simulink model "VCMGCM1962020b_v2"  (R2020b)
settings: Solver=FixedStepDiscrete  StartTime=0.0  StopTime=10.0  FixedStep=0.005  RelTol=1e-3  EnableMultiTasking=on
PreLoadFcn:
  | try, model_open; catch, disp('Error occurred while executing model pre-load callback: model_open.m'); disp('Please assure that the MATLAB working directory is set to the model directory before opening.'); end
InitFcn:
  | try, model_open; catch, end
undefined symbols (not defined in the file): Bridge, GCM, H, raptor_get_param_eval, raptor_get_safe_string, raptor_xcp_function
libraries: Blocks_lib x1165, Raptor_lib x665, simulink x62, VCM_lib x5
(part 23 of 23)

== stateflow chart VCMGCM1962020b_v2/Fgnd/Actuators/CAN/Drive Inverter/NMT Sequence ==
  state Init
    en: NMTStep= 1
    en:tmr=0;
    tmr++;
  state NMTSequenceActive
    state NMTStep2
      en: NMTStep= 2
      en: tmr = 0;
      du: tmr++;
    state NMTStep3
      en: NMTStep= 3
      en: tmr = 0;
      du: tmr++;
    state NMTStep4
      en: NMTStep= 4
      en: tmr = 0;
      du: tmr++;
    state NMTStep8
      en: NMTStep= 8;en: tmr = 0;
      du: tmr++;
    state NMTStep5
      en: NMTStep= 5;en: tmr = 0;
      du: tmr++;
    state NMTStep6
      en: NMTStep= 6;en: tmr = 0;
      du: tmr++;
    state NMTStep7
      en: NMTStep= 7;en: tmr = 0;
      du: tmr++;
    NMTStep8 -> NMTStep2 : [RunMode]
    NMTStep2 -> NMTStep5 [order 1] : [AutoStrEnbl && HV_On&& RunMode]
    NMTStep2 -> NMTStep3 [order 2] : [HV_On && tmr>NMTStateDly ]
    NMTStep3 -> NMTStep4 : [tmr>  NMTStateDly]
    NMTStep4 -> NMTStep5 : [tmr>  NMTStateDly && RunMode]
    NMTStep7 -> NMTStep8 : [tmr>  NMTStateDly]
    NMTStep5 -> NMTStep6 : [tmr>  NMTStateDly && !RunMode]
    NMTStep6 -> NMTStep7 : [tmr > NoComTm]
  note: Step2:
      | Nothing sent Wait HV
      | Step3:
      | VCU1_StateCmd = 0x0 (Off)
      | VCU2_EmTorqDmd = 0 Nm
      | VCU2_EmVelDmd = 0 Nm
      | Step4(1Frame):
      | NMT_StateDms_0x01 (operational)
      | TargetNode = 0x01
      | Step5 :
      | Enable Run mode, and apply torque
      | VCU1_StateCmd = 0x1 (RUN)
      | Step6:
      | VCU1_StateCmd = 0x0 (OFF)
      | Step7:
      | NMT_StateDmd = 0x02 (STOP)
      | NMT_TargetNode = 0x01
      | 1 frame
      | Step8: Stop VCU1/2 transmit
      |
      | Step 10: Error Reset
  state ErrorState
    en: NMTStep= 10
    en: tmr = 0;
    du: tmr++;
  note: Error reset
  (default) -> Init
  Init -> NMTStep2 : [tmr>NMTStateDly && InvrtrEnble]
  NMTSequenceActive -> Init [order 2] : [!InvrtrEnble]
  ErrorState -> NMTStep3 : [tmr>  NMTStateDly]
  NMTSequenceActive -> ErrorState [order 1] : [EM1StateAct==2 || (!EMxRcved && tmr > NoComTm)]
  data: tmr local double; NMTStateDly input double; EMxRcved input boolean; NoComTm input; HV_On input uint8 size=1; RunMode input boolean; NMTStep output uint8; EM1StateAct input boolean; InvrtrEnble input boolean; AutoStrEnbl input boolean

== stateflow chart VCMGCM1962020b_v2/Fgnd/Control/Other/Heater/Heater Pump ==
  state PUMP_ON
    en: Pump = 1
    state HEATER_ON
    state HEATER_OFF
      en: Tmr = 1
      du: Tmr ++
      ex: Tmr = 1
    (default) -> HEATER_ON
    HEATER_ON -> HEATER_OFF : [ !Heater ]
    HEATER_OFF -> HEATER_ON : [ Heater ]
  state PUMP_OFF
    en: Pump = 0
  (default) -> PUMP_OFF
  PUMP_OFF -> PUMP_ON : [ Enbl && Heater ]
  PUMP_ON -> PUMP_OFF : [ !Enbl || ...
      |   Tmr >= HoldTime ]
  data: Enbl input; Pump output boolean size=1; Tmr local uint16 size=1; Heater input; HoldTime input

== stateflow chart VCMGCM1962020b_v2/Fgnd/Control/PDU/High-Voltage Discharge Contactor/HV Discharge ==
  state ENABLE
    state DISCHARGE
      en: Cntr = 1
      en: Tmr = 1
      du: Tmr ++
    state FAULT
      en: Cntr = 0
      en: EvalDiag(1)
      en: Tmr = 1
      du: Tmr ++
    (default) -> DISCHARGE
    DISCHARGE -> FAULT : [ Tmr >= MxTime ]
    FAULT -> DISCHARGE : [ Tmr >= RetryWaitTime ]
  state DISABLE
    en: Cntr = 0
  state EvalDiag(status) [function]
  (default) -> DISABLE
  DISABLE -> ENABLE : [ Enbl ]
  ENABLE -> DISABLE : [ !Enbl ]
      | { EvalDiag(0) }
  data: status function_input; Cntr output boolean size=1; Tmr local uint16 size=1; Enbl input; MxTime input; RetryWaitTime input

== stateflow chart VCMGCM1962020b_v2/Fgnd/Control/Other/Other/FMWS/Chart ==
  (junction 11) -> (junction 13) : {FMWS_State_gear = 194 }
  (junction 3) -> (junction 11) [order 1] : [Drv == 1]
  (junction 25) -> (junction 3)
  (junction 3) -> (junction 15) [order 2] : [Ntrl == 1]
  (junction 15) -> (junction 17) : {FMWS_State_gear = 192 }
  (junction 44) -> (junction 25) [order 1] : [PrkBrk == 0]
  (junction 3) -> (junction 21) [order 3] : [Rev ==1]
  (junction 21) -> (junction 19) : {FMWS_State_gear = 196}
  (junction 30) -> (junction 36) : {FMWS_State_gear = 146 }
  (default) -> (junction 44)
  (junction 32) -> (junction 30) [order 1] : [Drv == 1]
  (junction 44) -> (junction 29) [order 2] : [PrkBrk ==1]
  (junction 29) -> (junction 32)
  (junction 32) -> (junction 40) [order 2] : [Ntrl == 1]
  (junction 40) -> (junction 39) : {FMWS_State_gear = 144 }
  (junction 32) -> (junction 43) [order 3] : [Rev ==1]
  (junction 43) -> (junction 42) : {FMWS_State_gear = 148}
  data: Drv input; Ntrl input; Rev input; PrkBrk input; FMWS_State_gear output

== stateflow chart VCMGCM1962020b_v2/Fgnd/Actuators/CAN/Charger/Config Msgs/Config Sequence/Config Sequence ==
  state WAIT
  state CONFIG
    en: Tmr1 = 1
    du: Tmr1 ++
    state TX617_A5
      en: Tx617_A5
      en: Tmr2 = 1
      du: Tmr2 ++
    state TX617_00
      en: Tx617_00
    (default) -> TX617_A5
    (junction 80) -> TX617_A5
    (junction 71) -> (junction 80)
    TX617_A5 -> (junction 69) : [ Tmr2 >= TxRate ]
    (junction 69) -> (junction 71) [order 2]
    (junction 69) -> TX617_00 [order 1] : [ ConfigComplete ]
  (default) -> WAIT
  WAIT -> CONFIG : [ hasChangedTo(ConfigPrompt, 1) ]
  CONFIG -> WAIT : [ Tmr1 >= MxTime ]
  TX617_00 -> WAIT
  data: ConfigPrompt input; ConfigComplete input; Tmr1 local uint16 size=1; Tmr2 local uint16 size=1; MxTime input; TxRate input
  events: Tx617_A5 output FUNCTION_CALL_EVENT; Tx617_00 output FUNCTION_CALL_EVENT

== stateflow chart VCMGCM1962020b_v2/Fgnd/Control/Modes/PRND Mode/PRND_Act ==
  (junction 5) -> (junction 17) : {PRND_Act_Out = 25}
  (junction 3) -> (junction 5) [order 1] : [PRND_In == 0]
  (junction 6) -> (junction 13) : {PRND_Act_Out = -125}
  (junction 3) -> (junction 6) [order 2] : [PRND_In == 1]
  (default) -> (junction 3)
  (junction 3) -> (junction 7) [order 3] : [PRND_In == 3]
  (junction 3) -> (junction 8) [order 4] : [PRND_In == 2]
  (junction 7) -> (junction 15) : {PRND_Act_Out = 125}
  (junction 8) -> (junction 19) : {PRND_Act_Out = 125}
  data: PRND_In input; PRND_Act_Out output

== stateflow chart VCMGCM1962020b_v2/Fgnd/Actuators/CAN/CCS Interface/Commands/Commands ==
  state WAIT_FOR_CABLE
    en: Step = 0.00
    en: Command = 2 %Standby
    en: EVTargetVoltage = 0
    en: EVTargetCurrent = 0
    en: DCChgCntr = 0
    en: DC_ContactorsState = 0
    en: BattIsoTestDsbl = 0
    en: ChgPortDCVoltHiDiagEnbl = 1
  state ON_BOARD_AC_CHARGING
    state NO_FAULT
      state CHARGING
        state WAIT_FOR_READY_TO_CHARGE
          en: Step = 1.00
          en: Command = 3 %Start
        state CHARGING
          en: Step = 1.01
          en: Command = 5 %Charge
        (default) -> WAIT_FOR_READY_TO_CHARGE
        WAIT_FOR_READY_TO_CHARGE -> ON_BOARD_AC_CHARGING.NO_FAULT.CHARGING.CHARGING : [ CurrentState == 8 ]
            | %Active_Ready To Charge
      state END_CHARGE
        en: Step = 1.02
        en: Command = 6 %End Charge
      (default) -> ON_BOARD_AC_CHARGING.NO_FAULT.CHARGING
      ON_BOARD_AC_CHARGING.NO_FAULT.CHARGING -> ON_BOARD_AC_CHARGING.NO_FAULT.END_CHARGE : [ !ChgMode ]
    state FAULT
      en: Step = 1.03
      en: Command = 2 %Standby
    (default) -> ON_BOARD_AC_CHARGING.NO_FAULT
    ON_BOARD_AC_CHARGING.NO_FAULT -> ON_BOARD_AC_CHARGING.FAULT : [ CurrentState == 12 ]
        | %Fault
    ON_BOARD_AC_CHARGING.FAULT -> (junction 265) : [ CurrentState == 0 || ...
        |   CurrentState == 1 || ...
        |   CurrentState == 15 || ...
        |   CurrentState == 16 || ...
        |   CurrentState == 17 ]
        | %Standby_*
    ON_BOARD_AC_CHARGING.NO_FAULT.END_CHARGE -> (junction 264) : [ CurrentState == 0 || ...
        |   CurrentState == 1 || ...
        |   CurrentState == 15 || ...
        |   CurrentState == 16 || ...
        |   CurrentState == 17 ]
        | %Standby_*
    (junction 265) -> (junction 264)
  state OFF_BOARD_DC_CHARGING
    state NO_FAULT
      state EVSE_PRECHARGE_AND_CHARGING
        state WAIT_FOR_READY_TO_PRECHARGE
          en: Step = 2.00
          en: Command = 3 %Start
        state PRECHARGE
          en: Step = 2.01
          en: Command = 4 %PreCharge
          en, du: EVTargetVoltage = HVBusVolt
          en: EVTargetCurrent = EVTargetCurrentPreChg
          en: ChgPortDCVoltHiDiagEnbl = 0
        state EVSE_PRECHARGED
          en: Step = 2.02
          en: Command = 5 %Charge
          en, du: EVTargetVoltage = HVBusVolt
          en: BattIsoTestDsbl = 1
          en: Tmr = 1; du: Tmr ++
        state CLOSE_DC_CHARGE_CONTACTORS
          en: Step = 2.03
          en: DCChgCntr = 1
          en, du: EVTargetVoltage = HVBusVolt
        state WAIT_FOR_ACTIVE_CHARGING
          en: Step = 2.04
          en: DC_ContactorsState = 1
        state RAMP_IN_CURRENT
          en: Step = 2.05
          en: EVTargetVoltage = ChgrDCVoltSetpt
          du: EVTargetCurrent = ...
          EVTargetCurrent + EVTargetCurrentRampInRate
        state NORMAL_CHARGING
          en: Step = 2.06
          en, du: EVTargetCurrent = ChgrDCCurLim
        (default) -> WAIT_FOR_READY_TO_PRECHARGE
        WAIT_FOR_READY_TO_PRECHARGE -> PRECHARGE : [ CurrentState == 6 ]
            | %Active_Ready for PreCharge
        PRECHARGE -> EVSE_PRECHARGED : [ ChgPortDCVoltMatch ]
        EVSE_PRECHARGED -> CLOSE_DC_CHARGE_CONTACTORS : [ ChgPortDCVoltMatch && ...
            |   DC_CloseContactorsRequest && ...
            |   Tmr >= BattIsoTestDsblTime ]
        CLOSE_DC_CHARGE_CONTACTORS -> WAIT_FOR_ACTIVE_CHARGING : [ DCChgCntrClosed ]
        WAIT_FOR_ACTIVE_CHARGING -> RAMP_IN_CURRENT : [ CurrentState == 9 ]
            | %Active_Charging
        RAMP_IN_CURRENT -> NORMAL_CHARGING : [ EVTargetCurrent >= ChgrDCCurLim ]
      state SHUTDOWN
        state RAMP_OUT_CURRENT
          en: Step = 2.07
          du: EVTargetCurrent = ...
          EVTargetCurrent + EVTargetCurrentRampOutRate
        state END_CHARGE
          en: Step = 2.08
          en: Command = 6 %End Charge
          en: EVTargetCurrent = 0
        state OPEN_DC_CHARGE_CONTACTORS
          en: Step = 2.09
          en: EVTargetVoltage = 0
          en: DCChgCntr = 0
          en: ChgPortDCVoltHiDiagEnbl = 1
        state WAIT_FOR_STANDBY
          en: Step = 2.10
          en: DC_ContactorsState = 0
          en: BattIsoTestDsbl = 0
        (default) -> RAMP_OUT_CURRENT
        RAMP_OUT_CURRENT -> OFF_BOARD_DC_CHARGING.NO_FAULT.SHUTDOWN.END_CHARGE : [ EVTargetCurrent <= 0 ]
        OFF_BOARD_DC_CHARGING.NO_FAULT.SHUTDOWN.END_CHARGE -> OFF_BOARD_DC_CHARGING.NO_FAULT.SHUTDOWN.OPEN_DC_CHARGE_CONTACTORS : [ !DC_CloseContactorsRequest ]
        OFF_BOARD_DC_CHARGING.NO_FAULT.SHUTDOWN.OPEN_DC_CHARGE_CONTACTORS -> OFF_BOARD_DC_CHARGING.NO_FAULT.SHUTDOWN.WAIT_FOR_STANDBY : [ DCChgCntrOpen && ...
            |   ChgPortDCVoltZero ]
      (default) -> EVSE_PRECHARGE_AND_CHARGING
      EVSE_PRECHARGE_AND_CHARGING -> SHUTDOWN : [ !ChgMode ]
    state FAULT
      state WAIT_FOR_CONTACTORS_OPEN_REQ
        en: Step = 2.11
        en: EVTargetCurrent = 0
      state WAIT_FOR_ZERO_CURRENT
        en: Step = 2.12
        en: Tmr = 1; du: Tmr ++
      state OPEN_DC_CHARGE_CONTACTORS
        en: Step = 2.13
        en: EVTargetVoltage = 0
        en: DCChgCntr = 0
        en: ChgPortDCVoltHiDiagEnbl = 1
      state WAIT_FOR_STANDBY
        en: Step = 2.14
        en: Command = 2 %Standby
        en: DC_ContactorsState = 0
        en: BattIsoTestDsbl = 0
      (default) -> WAIT_FOR_CONTACTORS_OPEN_REQ
      WAIT_FOR_CONTACTORS_OPEN_REQ -> WAIT_FOR_ZERO_CURRENT : [ !DC_CloseContactorsRequest ]
      WAIT_FOR_ZERO_CURRENT -> OFF_BOARD_DC_CHARGING.FAULT.OPEN_DC_CHARGE_CONTACTORS : [ ChgPortDCCurZero || ...
          |   Tmr >= ChgPortDCCurZeroMxTime ]
      OFF_BOARD_DC_CHARGING.FAULT.OPEN_DC_CHARGE_CONTACTORS -> OFF_BOARD_DC_CHARGING.FAULT.WAIT_FOR_STANDBY : [ DCChgCntrOpen && ...
          |   ChgPortDCVoltZero ]
    (default) -> OFF_BOARD_DC_CHARGING.NO_FAULT
    OFF_BOARD_DC_CHARGING.NO_FAULT.SHUTDOWN.WAIT_FOR_STANDBY -> (junction 281) : [ CurrentState == 0 || ...
        |   CurrentState == 1 || ...
        |   CurrentState == 15 || ...
        |   CurrentState == 16 || ...
        |   CurrentState == 17 ]
        | %Standby_*
    OFF_BOARD_DC_CHARGING.NO_FAULT -> OFF_BOARD_DC_CHARGING.FAULT : [ CurrentState == 12 ]
        | %Fault
    OFF_BOARD_DC_CHARGING.FAULT.WAIT_FOR_STANDBY -> (junction 281) : [ CurrentState == 0 || ...
        |   CurrentState == 1 || ...
        |   CurrentState == 15 || ...
        |   CurrentState == 16 || ...
        |   CurrentState == 17 ]
        | %Standby_*
  (default) -> WAIT_FOR_CABLE
  WAIT_FOR_CABLE -> ON_BOARD_AC_CHARGING [order 1] : [ ChgMode && ...
      |   CurrentState == 16 ]
      | %Standby_Cable Connected_Ready for Basic AC
  (junction 262) -> WAIT_FOR_CABLE
  WAIT_FOR_CABLE -> OFF_BOARD_DC_CHARGING [order 2] : [ ChgMode && ...
      |   CurrentState == 15 ]
      | %Standby_Cable Connected_Ready for HLC
  (junction 286) -> WAIT_FOR_CABLE
  (junction 264) -> (junction 262)
  (junction 281) -> (junction 286)
  data: ChgMode input; Step output double size=1; Command output uint8 size=1; EVTargetVoltage output double size=1; CurrentState input; EVTargetCurrent output double size=1; BattIsoTestDsbl output boolean size=1; DCChgCntr output boolean size=1; HVBusVolt input; ChgrDCVoltSetpt input; ChgrDCCurLim input; DC_CloseContactorsRequest input; ChgPortDCVoltMatch input; ChgPortDCVoltZero input; ChgPortDCCurZero input; DCChgCntrClosed input; DCChgCntrOpen input; DC_ContactorsState output boolean size=1; EVTargetCurrentPreChg input; BattIsoTestDsblTime input; EVTargetCurrentRampInRate input; EVTargetCurrentRampOutRate input; ChgPortDCCurZeroMxTime input; Tmr local double; ChgPortDCVoltHiDiagEnbl output boolean size=1
